simulink model "simmpc"  (Simulink 9.0)
settings: Solver=ode45  StartTime=0  StopTime=par.sim.Tstop  MaxStep=par.sim.Tstep  RelTol=1e-3  EnableMultiTasking=on
values from neighbouring files (symbols this model uses):
  alphas = pinv(X)*Y    [L2adaptivepredictor.m]
undefined symbols (not defined in the file or in its folder): inlvmat, mpc, predictionHorizon, predictorMat, wec, wecRealPlant
libraries: simulink x4
settings Model: LogicAnalyzerSignalOrdering=16dd2d14-8ec7-4c5d-8edb-c4853814402b,c13b3bd9-59af-45fd-871f-8fe12f09daf3,c1d8f7fc-636f-4d08-89ab-22a967bc3f49,540c2a49-8e05-4764-a29b-4d2006ad7b03,c655908f-e8fc-46d9-b655-4f5eab8146ef,1fcfe55d-85a2-4c68-9fe2-57e344af37ef,f1371f30-1a5b-431a-b1d1-69d0f6576f07,8fd6de23-e919-40ee-b8a8-5bcd4e916785,843b3b4a-383c-4e33-a49f-2e97cfb6bcb0,9188b340-1238-4cbc-a970-8c499a0eff54,224fac82-f9ba-4f20-9526-1cf49de6df85,94229721-9eb4-46fb-96b1-7eb35f4756a1,1d64066e-8085-4a65-8b92-701268a39d65  Creator=brekken  LastModifiedBy=ghorbanl
settings DataIOCC: LimitDataPoints=on
settings OptimizationCC: ExpressionDepthLimit=2147483647
settings DebuggingCC: SolverPrmCheckMsg=warning  FcnCallInpInsideContextMsg=warning  StateNameClashWarn=warning  StrictBusMsg=Warning
settings SFSimCC: SimParseCustomCode=off
settings GRTTargetCC: GeneratePreprocessorConditionals=Disable all  CombineOutputUpdateFcns=off  GRTInterface=on

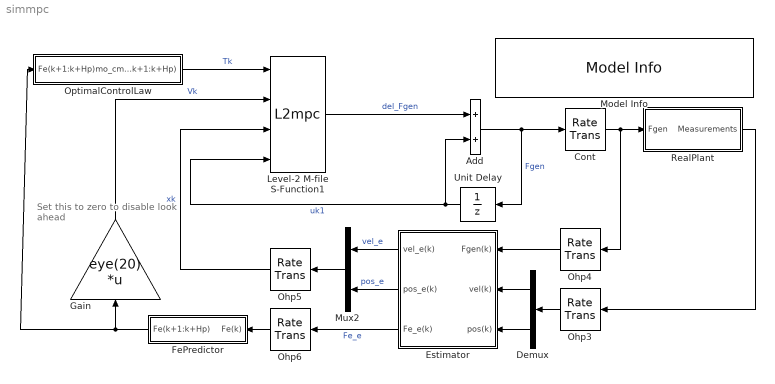
== system simmpc ==
  note: Set this to
      | zero to disable
      | look ahead
  Add : Sum
  Cont : RateTransition  Deterministic=off  OutPortSampleTime=0
  Demux : Demux  Outputs=2
  Estimator : Subsystem
  FePredictor : Subsystem
  Gain : Gain  Gain=eye(20)  Multiplication=Matrix(K*u)
  Level-2 M-file S-Function1 : M-S-Function  FunctionName=L2mpc  Parameters=mpc.Sx,mpc.Su1,mpc.Su, mpc.Hv, mpc.Q, mpc.R, mpc.MOConstraints, mpc.MVConstraints, mpc.MVRateConstraints, mpc.Ts  mask{Sx=mpc.Sx, Su1=mpc.Su1, Su=mpc.Su, Hv=mpc.Hv, Q=mpc.Q, R=mpc.R, MOConstraints=mpc.MOConstraints, MVConstraints=mpc.MVConstraints, MVRateConstraints=mpc.MVRateConstraints, Ts=mpc.Ts}
      mask prompts: MOConstraints "Measured output constraints ([low1 high1 low2 high2])"; MVConstraints "Manipulated variable constraints ([low1 high1])"; MVRateConstraints "Manipulated variable rate constraints ([low1 high1])"; Ts "Sample Time"
  Model Info : simulink/Model-Wide Utilities/Model Info  Frame=on  DisplayStringWithTags=|  HorizontalTextAlignment=Center  LeftAlignmentValue=0.5
      | MPC For Ocean Wave Energy
      | Created:  Ted Brekken, Sep. 2010
      | Version:  %<ModelVersion>
      | Modified:  %<ModifiedDate> by %<ModifiedBy>
  Mux2 : Mux  Inputs=2
  Ohp3 : RateTransition  Deterministic=off  OutPortSampleTime=wec.sys2dEstimator.Ts
  Ohp4 : RateTransition  Deterministic=off  OutPortSampleTime=wec.sys2dEstimator.Ts
  Ohp5 : RateTransition  Deterministic=off  OutPortSampleTime=mpc.Ts
  Ohp6 : RateTransition  Deterministic=off  OutPortSampleTime=mpc.Ts
  OptimalControlLaw : Subsystem
  RealPlant : Subsystem
  Unit Delay : UnitDelay  SampleTime=mpc.Ts
  wires:
  Level-2 M-file S-Function1/1 -> Add/1  "del_Fgen"
  Unit Delay/1 -> Add/2, Level-2 M-file S-Function1/4  "uk1"
  OptimalControlLaw/1(mo_cmd(k+1:k+Hp)) -> Level-2 M-file S-Function1/1  "Tk"
  Cont/1 -> RealPlant/1(Fgen), Ohp4/1
  Ohp4/1 -> Estimator/1(Fgen(k))
  Demux/1 -> Estimator/2(vel(k))
  Demux/2 -> Estimator/3(pos(k))
  Ohp3/1 -> Demux/1
  Mux2/1 -> Ohp5/1
  Estimator/1(vel_e(k)) -> Mux2/1  "vel_e"
  Estimator/2(pos_e(k)) -> Mux2/2  "pos_e"
  Estimator/3(Fe_e(k)) -> Ohp6/1  "Fe_e"
  Ohp6/1 -> FePredictor/1(Fe(k))
  FePredictor/1(Fe(k+1:k+Hp)) -> OptimalControlLaw/1(Fe(k+1:k+Hp)), Gain/1
  Add/1 -> Unit Delay/1, Cont/1  "Fgen"
  RealPlant/1(Measurements) -> Ohp3/1
  Ohp5/1 -> Level-2 M-file S-Function1/3  "xk"
  Gain/1 -> Level-2 M-file S-Function1/2  "Vk"

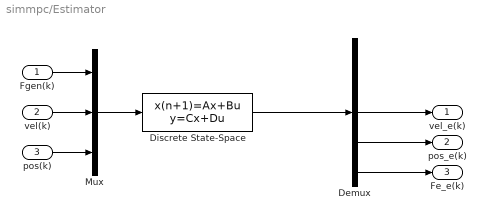
== system simmpc/Estimator ==
  Fgen(k) : Inport
  vel(k) : Inport  Port=2
  pos(k) : Inport  Port=3
  Demux : Demux  Outputs=5
  Discrete State-Space : DiscreteStateSpace  A=wec.sys2dEstimator.a  B=wec.sys2dEstimator.b  C=wec.sys2dEstimator.c  D=wec.sys2dEstimator.d  SampleTime=wec.sys2dEstimator.Ts
  Mux : Mux  Inputs=3
  vel_e(k) : Outport
  pos_e(k) : Outport  Port=2
  Fe_e(k) : Outport  Port=3
  wires:
  Fgen(k)/1 -> Mux/1
  vel(k)/1 -> Mux/2
  pos(k)/1 -> Mux/3
  Mux/1 -> Discrete State-Space/1
  Discrete State-Space/1 -> Demux/1
  Demux/3 -> vel_e(k)/1
  Demux/4 -> pos_e(k)/1
  Demux/5 -> Fe_e(k)/1

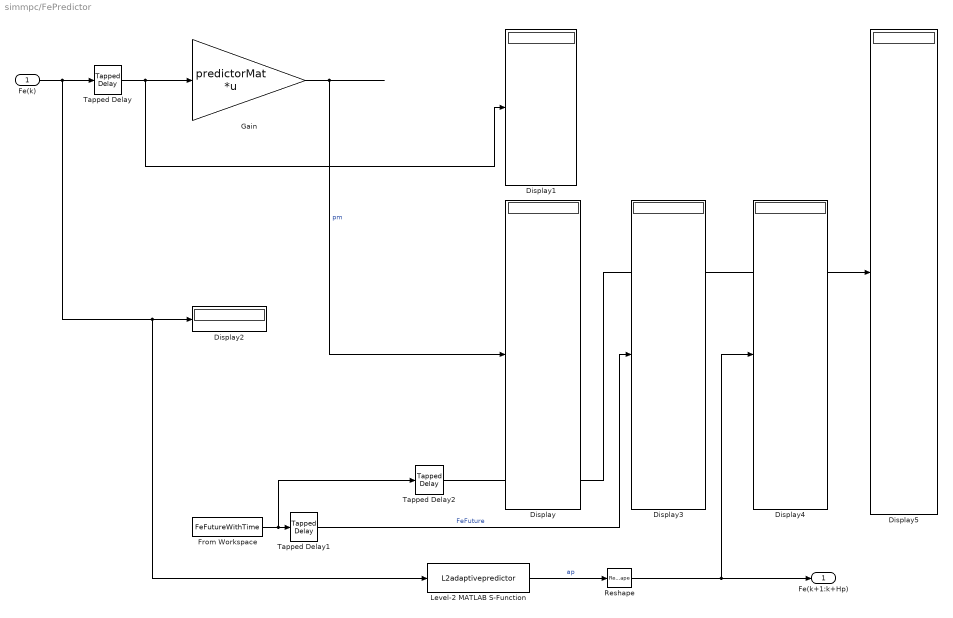
== system simmpc/FePredictor ==
  Fe(k) : Inport
  Display{,1..5} (6 alike) : Display
  From Workspace : FromWorkspace  VariableName=FeFutureWithTime  OutputAfterFinalValue=Setting to zero
  Gain : Gain  Gain=predictorMat  Multiplication=Matrix(K*u)
  Level-2 MATLAB S-Function : M-S-Function  FunctionName=L2adaptivepredictor  Parameters=20, 100, 10
  Reshape : Reshape
  Tapped Delay : simulink/Discrete/Tapped Delay  vinit=0.0  samptime=mpc.Ts  NumDelays=length(alphas)-1  DelayOrder=Oldest  includeCurrent=on
  Tapped Delay1 : simulink/Discrete/Tapped Delay  vinit=0.0  samptime=mpc.Ts  NumDelays=predictionHorizon-1  DelayOrder=Oldest  includeCurrent=on
  Tapped Delay2 : simulink/Discrete/Tapped Delay  vinit=0.0  samptime=mpc.Ts  NumDelays=29  DelayOrder=Oldest  includeCurrent=on
  Fe(k+1:k+Hp) : Outport
  wires:
  Gain/1 -> Display/1  "pm"
  Tapped Delay/1 -> Gain/1, Display1/1
  From Workspace/1 -> Tapped Delay1/1, Tapped Delay2/1
  Tapped Delay1/1 -> Display3/1  "FeFuture"
  Fe(k)/1 -> Tapped Delay/1, Display2/1, Level-2 MATLAB S-Function/1
  Level-2 MATLAB S-Function/1 -> Reshape/1  "ap"
  Reshape/1 -> Display4/1, Fe(k+1:k+Hp)/1
  Tapped Delay2/1 -> Display5/1

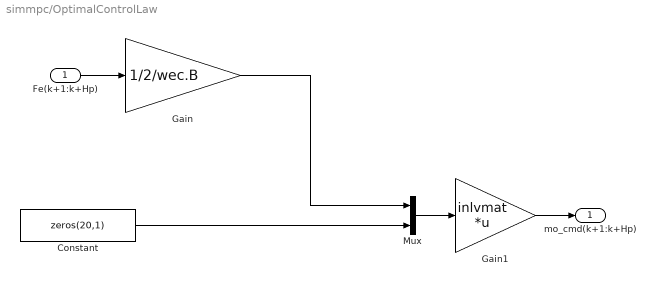
== system simmpc/OptimalControlLaw ==
  Fe(k+1:k+Hp) : Inport
  Constant : Constant  Value=zeros(20,1)
  Gain : Gain  Gain=1/2/wec.B
  Gain1 : Gain  Gain=inlvmat  Multiplication=Matrix(K*u)
  Mux : Mux  Inputs=2
  mo_cmd(k+1:k+Hp) : Outport
  wires:
  Fe(k+1:k+Hp)/1 -> Gain/1
  Gain/1 -> Mux/1
  Mux/1 -> Gain1/1
  Constant/1 -> Mux/2
  Gain1/1 -> mo_cmd(k+1:k+Hp)/1

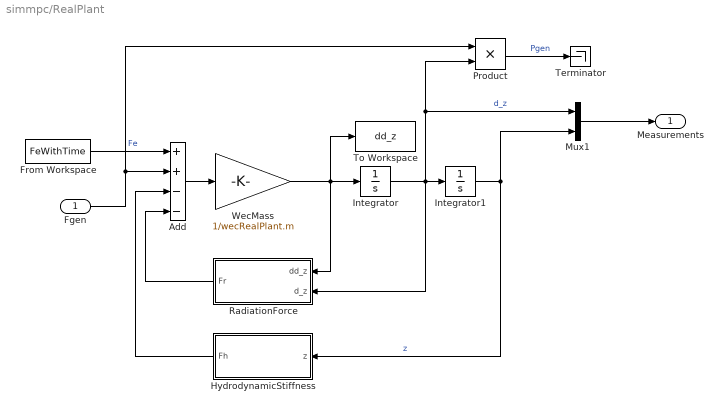
== system simmpc/RealPlant ==
  Fgen : Inport
  Add : Sum  Inputs=++--
  From Workspace : FromWorkspace  VariableName=FeWithTime  SampleTime=0
  HydrodynamicStiffness : Subsystem
  Integrator : Integrator
  Integrator1 : Integrator
  Mux1 : Mux  Inputs=2
  Product : Product  RndMeth=Zero
  RadiationForce : Subsystem
  Terminator : Terminator
  To Workspace : ToWorkspace  VariableName=dd_z  SaveFormat=Structure  SampleTime=-1
  WecMass : Gain  Gain=1/wecRealPlant.m
  Measurements : Outport
  wires:
  Integrator/1 -> Integrator1/1, RadiationForce/2(d_z), Mux1/1, Product/2  "d_z"
  WecMass/1 -> Integrator/1, RadiationForce/1(dd_z), To Workspace/1
  Integrator1/1 -> HydrodynamicStiffness/1(z), Mux1/2  "z"
  Add/1 -> WecMass/1
  RadiationForce/1(Fr) -> Add/4
  HydrodynamicStiffness/1(Fh) -> Add/3
  Mux1/1 -> Measurements/1
  From Workspace/1 -> Add/1  "Fe"
  Fgen/1 -> Add/2, Product/1
  Product/1 -> Terminator/1  "Pgen"

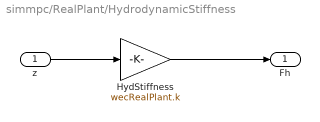
== system simmpc/RealPlant/HydrodynamicStiffness ==
  z : Inport
  HydStiffness : Gain  Gain=wecRealPlant.k
  Fh : Outport
  wires:
  z/1 -> HydStiffness/1
  HydStiffness/1 -> Fh/1

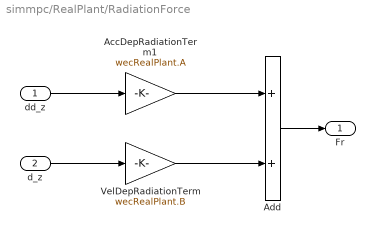
== system simmpc/RealPlant/RadiationForce ==
  dd_z : Inport
  d_z : Inport  Port=2
  AccDepRadiationTerm1 : Gain  Gain=wecRealPlant.A
  Add : Sum
  VelDepRadiationTerm : Gain  Gain=wecRealPlant.B
  Fr : Outport
  wires:
  d_z/1 -> VelDepRadiationTerm/1
  dd_z/1 -> AccDepRadiationTerm1/1
  AccDepRadiationTerm1/1 -> Add/1
  VelDepRadiationTerm/1 -> Add/2
  Add/1 -> Fr/1
